simulink model "sol1_2_combined"  (R2021b)
settings: Solver=VariableStepAuto  StartTime=0.0  StopTime=1  RelTol=1e-3
PreLoadFcn:
  | initModelData
values from neighbouring files (symbols this model uses):
  B = Bm+(Kb*Km/R)    (= 0.0149065789474)    [MyData_for_1_and_2.m]    (also in MyData_for_3_4_and_5.m; MyData_for_5_and_6.m)
  Bm = 4e-4    (= 0.0004)    [MyData_for_1_and_2.m]    (also in MyData_for_3_4_and_5.m; MyData_for_5_and_6.m)
  Jm = 5.5e-4    (= 0.00055)    [MyData_for_1_and_2.m]    (also in MyData_for_3_4_and_5.m; MyData_for_5_and_6.m)
  Kb = 0.105    [MyData_for_1_and_2.m]    (also in MyData_for_3_4_and_5.m; MyData_for_5_and_6.m)
  Km = 0.105    [MyData_for_1_and_2.m]    (also in MyData_for_3_4_and_5.m; MyData_for_5_and_6.m)
  L = 0.9e-3    (= 0.0009)    [MyData_for_1_and_2.m]    (also in MyData_for_3_4_and_5.m; MyData_for_5_and_6.m)
  r = 156    [MyData_for_1_and_2.m]    (also in MyData_for_3_4_and_5.m; MyData_for_5_and_6.m)
  R = 0.76    [MyData_for_1_and_2.m]    (also in MyData_for_3_4_and_5.m; MyData_for_5_and_6.m)
settings Model: Creator=esdan  LastModifiedBy=munir
settings SolverCC: AlgebraicLoopSolver=TrustRegion
settings DebuggingCC: SFMachineParentedDataDiag=warning

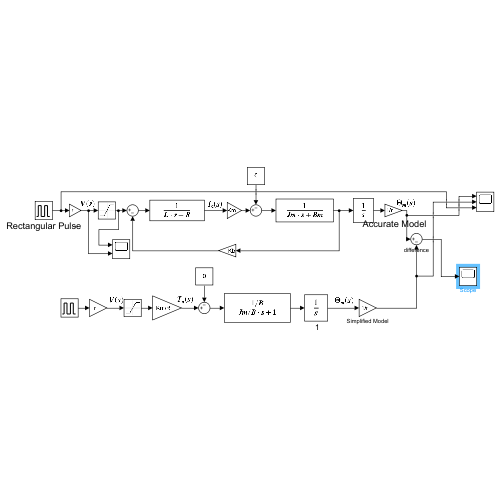
[thumbnail: Simulink's stored preview of the top-level diagram]
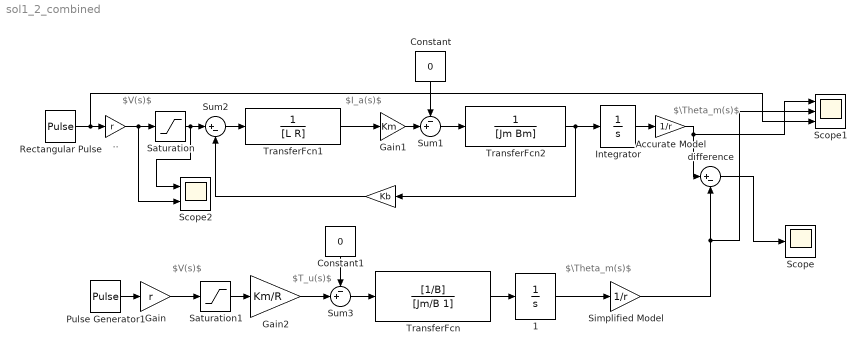
== system sol1_2_combined ==
  note: $I_a(s)$
  note: $\Theta_m(s)$
  note: $V(s)$
  note: $T_u(s)$
  note: $V(s)$
  note: $\Theta_m(s)$
  " " : Gain  Gain=Kb
  " .." : Gain  Gain=r
  " 1" : Integrator
  " Accurate Model" : Gain  Gain=1/r
  Constant : Constant  Value=0
  Constant1 : Constant  Value=0
  Gain : Gain  Gain=r
  Gain1 : Gain  Gain=Km
  Gain2 : Gain  Gain=Km/R
  Integrator : Integrator
  Pulse Generator1 : DiscretePulseGenerator  PulseType=Time based  Period=1  PulseWidth=50
  Rectangular Pulse : DiscretePulseGenerator  PulseType=Time based  Period=1  PulseWidth=50
  Saturation : Saturate  UpperLimit=35  LowerLimit=-35
  Saturation1 : Saturate  UpperLimit=35  LowerLimit=-35
  Scope : Scope
  Scope1 : Scope  NumInputPorts=3
  Scope2 : Scope  NumInputPorts=2
  Simplified Model : Gain  Gain=1/r
  Sum1 : Sum  Inputs=-+|
  Sum2 : Sum  Inputs=|+-
  Sum3 : Sum  Inputs=-+|
  TransferFcn : TransferFcn  Numerator=[1/B]  Denominator=[Jm/B 1]
  TransferFcn1 : TransferFcn  Denominator=[L R]
  TransferFcn2 : TransferFcn  Denominator=[Jm Bm]
  difference : Sum  Inputs=|+-
  wires:
  TransferFcn1/1 -> Gain1/1
  Sum2/1 -> TransferFcn1/1
  TransferFcn2/1 -> " "/1, Integrator/1
  " "/1 -> Sum2/2
  Saturation/1 -> Scope2/1, Sum2/1
  Sum1/1 -> TransferFcn2/1
  Gain1/1 -> Sum1/2
  Constant/1 -> Sum1/1
  " .."/1 -> Scope2/2, Saturation/1
  " Accurate Model"/1 -> difference/1, Scope1/1
  Integrator/1 -> " Accurate Model"/1
  Rectangular Pulse/1 -> Scope1/3, " .."/1
  Pulse Generator1/1 -> Gain/1
  Gain/1 -> Saturation1/1
  Sum3/1 -> TransferFcn/1
  TransferFcn/1 -> " 1"/1
  Saturation1/1 -> Gain2/1
  Gain2/1 -> Sum3/2
  " 1"/1 -> Simplified Model/1
  Constant1/1 -> Sum3/1
  Simplified Model/1 -> Scope1/2, difference/2
  difference/1 -> Scope/1
